simulink model "Final_simulation_with_copensation_and_filters"  (R2015a)
settings: Solver=ode23t  SolverMode=SingleTasking  StartTime=0.0  StopTime=0.1  RelTol=1e-3
libraries: powerlib x42, powerlib_meascontrol x1
settings Model: CovSFcnEnable=off  Creator=sebitosi  LastModifiedBy=noni
settings OptimizationCC: BlockReduction=off  BooleanDataType=off
settings DebuggingCC: SaveWithParameterizedLinksMsg=none  UnderspecifiedInitializationDetection=Classic  MergeDetectMultiDrivingBlocksExec=none  SignalResolutionControl=TryResolveAllWithWarning
settings HardwareCC: TargetUnknown=on

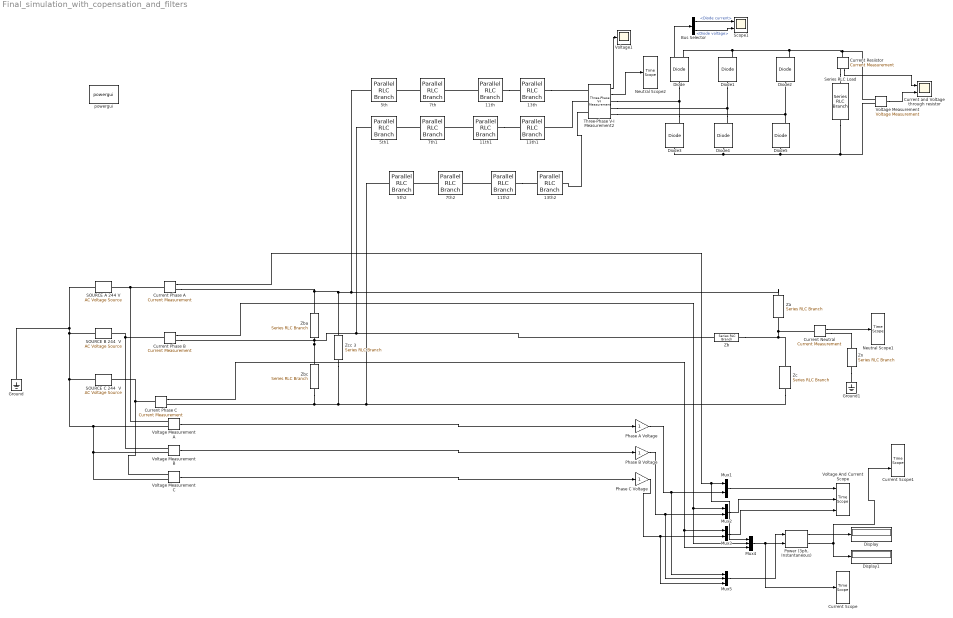
== system Final_simulation_with_copensation_and_filters ==
  " SOURCE B 244  V" : powerlib/Electrical Sources/AC Voltage Source  Amplitude=244  Phase=-120  Frequency=50  SampleTime=0  Measurements=None
  " Voltage Measurement" : powerlib/Measurements/Voltage Measurement  PhasorSimulation=off  OutputType=Complex  PSBequivalent=0
  11th : powerlib/Elements/Parallel RLC Branch  LConnTagsString=a  RConnTagsString=__new0  BranchType=LC  Resistance=1  Inductance=4.7e-3  SetiL0=off  InitialCurrent=0  Capacitance=17.8e-6  Setx0=off  InitialVoltage=0  Measurements=None
  11th1 : powerlib/Elements/Parallel RLC Branch  LConnTagsString=a  RConnTagsString=__new0  BranchType=LC  Resistance=1  Inductance=4.7e-3  SetiL0=off  InitialCurrent=0  Capacitance=17.8e-6  Setx0=off  InitialVoltage=0  Measurements=None
  11th2 : powerlib/Elements/Parallel RLC Branch  LConnTagsString=a  RConnTagsString=__new0  BranchType=LC  Resistance=1  Inductance=4.7e-3  SetiL0=off  InitialCurrent=0  Capacitance=17.8e-6  Setx0=off  InitialVoltage=0  Measurements=None
  13th : powerlib/Elements/Parallel RLC Branch  LConnTagsString=a  RConnTagsString=__new0  BranchType=LC  Resistance=1  Inductance=4.7e-3  SetiL0=off  InitialCurrent=0  Capacitance=12.75e-6  Setx0=off  InitialVoltage=0  Measurements=None
  13th1 : powerlib/Elements/Parallel RLC Branch  LConnTagsString=a  RConnTagsString=__new0  BranchType=LC  Resistance=1  Inductance=4.7e-3  SetiL0=off  InitialCurrent=0  Capacitance=12.75e-6  Setx0=off  InitialVoltage=0  Measurements=None
  13th2 : powerlib/Elements/Parallel RLC Branch  LConnTagsString=a  RConnTagsString=__new0  BranchType=LC  Resistance=1  Inductance=4.7e-3  SetiL0=off  InitialCurrent=0  Capacitance=12.75e-6  Setx0=off  InitialVoltage=0  Measurements=None
  5th : powerlib/Elements/Parallel RLC Branch  LConnTagsString=a  RConnTagsString=__new0  BranchType=LC  Resistance=1  Inductance=4.7e-3  SetiL0=off  InitialCurrent=0  Capacitance=86.2e-6  Setx0=off  InitialVoltage=0  Measurements=None
  5th1 : powerlib/Elements/Parallel RLC Branch  LConnTagsString=a  RConnTagsString=__new0  BranchType=LC  Resistance=1  Inductance=4.7e-3  SetiL0=off  InitialCurrent=0  Capacitance=86.2e-6  Setx0=off  InitialVoltage=0  Measurements=None
  5th2 : powerlib/Elements/Parallel RLC Branch  LConnTagsString=a  RConnTagsString=__new0  BranchType=LC  Resistance=1  Inductance=4.7e-3  SetiL0=off  InitialCurrent=0  Capacitance=86.2e-6  Setx0=off  InitialVoltage=0  Measurements=None
  7th : powerlib/Elements/Parallel RLC Branch  LConnTagsString=a  RConnTagsString=__new0  BranchType=LC  Resistance=1  Inductance=4.7e-3  SetiL0=off  InitialCurrent=0  Capacitance=44e-6  Setx0=off  InitialVoltage=0  Measurements=None
  7th1 : powerlib/Elements/Parallel RLC Branch  LConnTagsString=a  RConnTagsString=__new0  BranchType=LC  Resistance=1  Inductance=4.7e-3  SetiL0=off  InitialCurrent=0  Capacitance=44e-6  Setx0=off  InitialVoltage=0  Measurements=None
  7th2 : powerlib/Elements/Parallel RLC Branch  LConnTagsString=a  RConnTagsString=__new0  BranchType=LC  Resistance=1  Inductance=4.7e-3  SetiL0=off  InitialCurrent=0  Capacitance=44e-6  Setx0=off  InitialVoltage=0  Measurements=None
  Bus Selector : BusSelector  OutputSignals=Diode current,Diode voltage
  Current Neutral : powerlib/Measurements/Current Measurement  PhasorSimulation=off  OutputType=Complex  PSBequivalent=0
  Current Phase A : powerlib/Measurements/Current Measurement  PhasorSimulation=off  OutputType=Complex  PSBequivalent=0
  Current Phase B : powerlib/Measurements/Current Measurement  PhasorSimulation=off  OutputType=Complex  PSBequivalent=0
  Current Phase C : powerlib/Measurements/Current Measurement  PhasorSimulation=off  OutputType=Complex  PSBequivalent=0
  Current Resiistor : powerlib/Measurements/Current Measurement  PhasorSimulation=off  OutputType=Complex  PSBequivalent=0
  Current Scope : TimeScope
  Current Scope1 : TimeScope  NumInputPorts=2
  Current and Voltage through resistor : Scope  NumInputPorts=2
      settings: YMin=-5~-5  YMax=5~5  SaveName=Load_voltage
  Diode{,1..5} (6 alike) : powerlib/Power Electronics/Diode  Ron=0.001  Lon=0  Vf=0.8  IC=0  UseSnubber=off  Rs=500  Cs=250e-9  Measurements=on
  Display : Display
  Display1 : Display
  Ground : powerlib/Elements/Ground  LConnTagsString=a
  Ground1 : powerlib/Elements/Ground  LConnTagsString=a
  Mux1 : Mux  Inputs=2
  Mux2 : Mux  Inputs=2
  Mux3 : Mux  Inputs=2
  Mux4 : Mux  Inputs=3
  Mux5 : Mux  Inputs=3
  Neutral Scope1 : TimeScope
  Neutral Scope2 : TimeScope
  Phase A Voltage : Gain
  Phase B Voltage : Gain
  Phase C Voltage : Gain
  "Power (3ph, Instantaneous)" : powerlib_meascontrol/Measurements/Power (3ph, Instantaneous)
  SOURCE A 244 V : powerlib/Electrical Sources/AC Voltage Source  Amplitude=244  Phase=0  Frequency=50  SampleTime=0  Measurements=None
  "SOURCE C 244  V " : powerlib/Electrical Sources/AC Voltage Source  Amplitude=244  Phase=120  Frequency=50  SampleTime=0  Measurements=None
  Scope1 : Scope  NumInputPorts=2
      settings: YMin=-5~-5  YMax=5~5  SaveName=Load_voltage1
  Series RLC Load : powerlib/Elements/Series RLC Branch  LConnTagsString=__new0  RConnTagsString=__new0  BranchType=R  Resistance=1  Inductance=1e-3  SetiL0=off  InitialCurrent=0  Capacitance=1e-6  Setx0=off  InitialVoltage=0  Measurements=None
  Three-Phase V-I Measurement2 : powerlib/Measurements/Three-Phase V-I Measurement  VoltageMeasurement=phase-to-ground  SetLabelV=off  LabelV=Vabc  Vpu=off  VpuLL=off  CurrentMeasurement=yes  SetLabelI=off  LabelI=Iabc  Ipu=off  Pbase=100e6  Vbase=500e3  OutputType=Complex  PhasorSimulation=off  PSBequivalent=0
  Voltage And Current Scope : TimeScope  NumInputPorts=3
  Voltage Measurement A : powerlib/Measurements/Voltage Measurement  PhasorSimulation=off  OutputType=Complex  PSBequivalent=0
  Voltage Measurement B : powerlib/Measurements/Voltage Measurement  PhasorSimulation=off  OutputType=Complex  PSBequivalent=0
  Voltage Measurement C : powerlib/Measurements/Voltage Measurement  PhasorSimulation=off  OutputType=Complex  PSBequivalent=0
  Voltage1 : Scope
      settings: SaveName=ScopeData3
  "Za " : powerlib/Elements/Series RLC Branch  LConnTagsString=__new0  RConnTagsString=__new0  BranchType=RL  Resistance=0.34  Inductance=0.5729e-3  SetiL0=off  InitialCurrent=0  Capacitance=1e-6  Setx0=off  InitialVoltage=0  Measurements=None
  "Zb " : powerlib/Elements/Series RLC Branch  LConnTagsString=__new0  RConnTagsString=__new0  BranchType=RL  Resistance=0.37  Inductance=0.7e-3  SetiL0=off  InitialCurrent=0  Capacitance=0  Setx0=off  InitialVoltage=0  Measurements=None
  Zba : powerlib/Elements/Series RLC Branch  LConnTagsString=__new0  RConnTagsString=__new0  BranchType=RC  Resistance=0.1  Inductance=0.7e-3  SetiL0=off  InitialCurrent=0  Capacitance=1.5e-3  Setx0=off  InitialVoltage=0  Measurements=None
  Zbc : powerlib/Elements/Series RLC Branch  LConnTagsString=__new0  RConnTagsString=__new0  BranchType=RC  Resistance=0.1  Inductance=0.7e-3  SetiL0=off  InitialCurrent=0  Capacitance=0.8e-3  Setx0=off  InitialVoltage=0  Measurements=None
  Zc : powerlib/Elements/Series RLC Branch  LConnTagsString=__new0  RConnTagsString=__new0  BranchType=RL  Resistance=0.36  Inductance=0.541e-3  SetiL0=off  InitialCurrent=0  Capacitance=7.96366e-4  Setx0=off  InitialVoltage=0  Measurements=None
  Zcc 3 : powerlib/Elements/Series RLC Branch  LConnTagsString=__new0  RConnTagsString=__new0  BranchType=RC  Resistance=0.1  Inductance=0.7e-3  SetiL0=off  InitialCurrent=0  Capacitance=1.1e-3  Setx0=off  InitialVoltage=0  Measurements=None
  Zn : powerlib/Elements/Series RLC Branch  LConnTagsString=__new0  RConnTagsString=__new0  BranchType=R  Resistance=8.8e-4  Inductance=2.58213e-4  SetiL0=off  InitialCurrent=0  Capacitance=1e-6  Setx0=off  InitialVoltage=0  Measurements=None
  powergui : powerlib/powergui  Priority=1  SimulationMode=Continuous  SolverType=Tustin  SampleTime=50e-6  frequency=60  SPID=off  DisableSnubberDevices=off  DisableRonSwitches=off  DisableVfSwitches=off  SwTol=0  DisplayEquations=off  Interpol=off  methode=off  Ts=100  FunctionMessages=off  echomessages=off  HookPort=off  EnableUseOfTLC=off  x0status=blocks  frequencyindice=0  Pbase=100e6  ErrMax=1e-4  Iterations=50  UnitsV=kV  UnitsW=MW  buscounter=0  RestoreLinks=warning  ResistiveCurrentMeasurement=off  Frange=[0:2:500]  Ylog=off  Xlog=off  ShowGrid=off  save=off  variable=ZData  structure=currents  ZoomFFT=off  StartTime=0.0  cycles=1  DisplayStyle=1  fundamental=50  FreqAxis=on  MaxFrequency=1000  frequencyindicesteady=1  RmsSteady=1  display=off
  wires:
  Mux1/1 -> Voltage And Current Scope/1
  Voltage Measurement C/1 -> Phase C Voltage/1
  Voltage Measurement B/1 -> Phase B Voltage/1
  Phase A Voltage/1 -> Mux5/1, Mux1/2
  Phase B Voltage/1 -> Mux5/2, Mux2/2
  Phase C Voltage/1 -> Mux3/2, Mux5/3
  Mux2/1 -> Voltage And Current Scope/2
  Mux3/1 -> Voltage And Current Scope/3
  Current Phase A/1 -> Mux4/1, Mux1/1
  Current Phase C/1 -> Mux4/3, Mux3/1
  Current Phase B/1 -> Mux4/2, Mux2/1
  Voltage Measurement A/1 -> Phase A Voltage/1
  Mux4/1 -> "Power (3ph, Instantaneous)"/2, Current Scope/1
  Current Neutral/1 -> Neutral Scope1/1
  Mux5/1 -> "Power (3ph, Instantaneous)"/1
  "Power (3ph, Instantaneous)"/1 -> Display/1
  "Power (3ph, Instantaneous)"/2 -> Display1/1, Current Scope1/2
  Diode/1 -> Bus Selector/1
  " Voltage Measurement"/1 -> Current and Voltage through resistor/2
  Current Resiistor/1 -> Current and Voltage through resistor/1
  Bus Selector/1 -> Scope1/1  "<Diode current>"
  Bus Selector/2 -> Scope1/2  "<Diode voltage>"
  Three-Phase V-I Measurement2/2 -> Neutral Scope2/1
  Three-Phase V-I Measurement2/1 -> Voltage1/1
  connections:
  Voltage Measurement A/LConn1 -- Current Phase A/LConn1 -- SOURCE A 244 V/RConn1
  Voltage Measurement C/LConn1 -- "SOURCE C 244  V "/RConn1 -- Current Phase C/LConn1
  Voltage Measurement C/LConn2 -- Voltage Measurement B/LConn2 -- Voltage Measurement A/LConn2 -- Ground/LConn1 -- SOURCE A 244 V/LConn1 -- " SOURCE B 244  V"/LConn1 -- "SOURCE C 244  V "/LConn1
  "Zb "/RConn1 -- Zc/RConn1 -- Current Neutral/LConn1 -- "Za "/RConn1
  Zn/RConn1 -- Ground1/LConn1
  Voltage Measurement B/LConn1 -- " SOURCE B 244  V"/RConn1 -- Current Phase B/LConn1
  Diode3/RConn1 -- Diode/LConn1 -- Three-Phase V-I Measurement2/RConn1
  Diode4/RConn1 -- Diode1/LConn1 -- Three-Phase V-I Measurement2/RConn2
  Diode2/RConn1 -- Current Resiistor/LConn1 -- " Voltage Measurement"/LConn1 -- Diode/RConn1 -- Diode1/RConn1
  Diode5/LConn1 -- Series RLC Load/RConn1 -- " Voltage Measurement"/LConn2 -- Diode3/LConn1 -- Diode4/LConn1
  Three-Phase V-I Measurement2/RConn3 -- Diode5/RConn1 -- Diode2/LConn1
  Current Resiistor/RConn1 -- Series RLC Load/LConn1
  Current Neutral/RConn1 -- Zn/LConn1
  Current Phase B/RConn1 -- 5th1/LConn1 -- "Zb "/LConn1 -- Zbc/LConn1 -- Zba/RConn1
  Current Phase A/RConn1 -- "Za "/LConn1 -- 5th/LConn1 -- Zcc 3/RConn1 -- Zba/LConn1
  Zcc 3/LConn1 -- 5th2/LConn1 -- Zc/LConn1 -- Zbc/RConn1 -- Current Phase C/RConn1
  11th/LConn1 -- 7th/RConn1
  7th/LConn1 -- 5th/RConn1
  13th/RConn1 -- Three-Phase V-I Measurement2/LConn1
  11th/RConn1 -- 13th/LConn1
  Three-Phase V-I Measurement2/LConn3 -- 13th2/RConn1
  11th1/LConn1 -- 7th1/RConn1
  11th1/RConn1 -- 13th1/LConn1
  Three-Phase V-I Measurement2/LConn2 -- 13th1/RConn1
  7th1/LConn1 -- 5th1/RConn1
  7th2/LConn1 -- 5th2/RConn1
  11th2/RConn1 -- 13th2/LConn1
  11th2/LConn1 -- 7th2/RConn1
